simulink model "CSTR_mpc8_simulink"  (R2023b)
settings: Solver=VariableStepAuto  StartTime=0.0  StopTime=10.0  RelTol=1e-3
libraries: mpclib x1, cstblocks x1
settings Model: Creator=epepe  LastModifiedBy=epepe

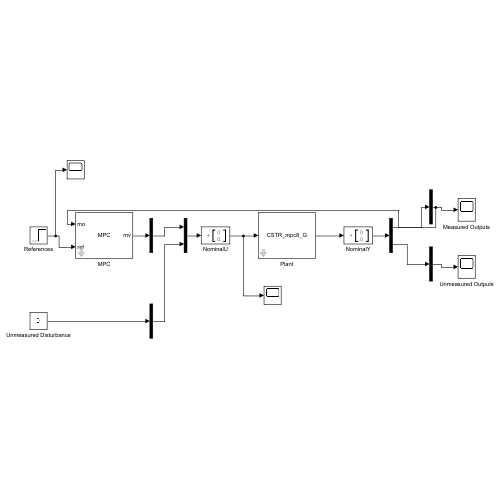
[thumbnail: Simulink's stored preview of the top-level diagram]
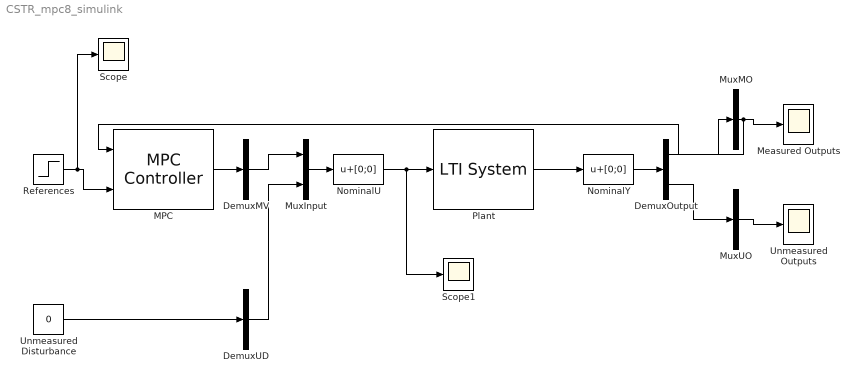
== system CSTR_mpc8_simulink ==
  DemuxMV : Demux  Outputs=1
  DemuxOutput : Demux  Outputs=2
  DemuxUD : Demux  Outputs=1
  MPC : mpclib/MPC Controller  SCDEnableBlockLinearizationSpecification=on  mpcobj=CSTR_mpc8_C  is_multiple=0  enable_value=0  return_u0=off  updateMPCinCallerWorkspace=on  md_inport=off  mv_inport=off  uref_inport=off  return_cost=off  return_mvseq=off  return_qpstatus=off  return_xseq=off  return_state=off  return_ovseq=off  state_inport=off  umin_inport=off  umax_inport=off  ymin_inport=off  ymax_inport=off  cc_inport=off  ywt_inport=off  uwt_inport=off  duwt_inport=off  rhoeps_inport=off  pm_inport=off  MaximumP=10  HorizonChoice=FixedHorizon  n_ts=0.5  n_p=15  n_mv=1  n_md=0  n_ud=1  n_mo=1  n_uo=1  BlockDataType=double  SampleTimeInherited=off  switch_inport=off
  Measured Outputs : Scope
  MuxInput : Mux  Inputs=2
  MuxMO : Mux  Inputs=1
  MuxUO : Mux  Inputs=1
  NominalU : Bias  Bias=[0;0]
  NominalY : Bias  Bias=[0;0]
  Plant : cstblocks/LTI System  sys=CSTR_mpc8_G  IC=[]  PadeOrder=0
  References : Step  Time=5  Before=[0;0]  After=[2;0]
  Scope : Scope
  Scope1 : Scope
  Unmeasured Disturbance : Constant  Value=0
  Unmeasured Outputs : Scope
  wires:
  References/1 -> Scope/1, MPC/2
  Plant/1 -> NominalY/1
  NominalY/1 -> DemuxOutput/1
  MuxMO/1 -> MPC/1, Measured Outputs/1
  MuxUO/1 -> Unmeasured Outputs/1
  DemuxOutput/1 -> MuxMO/1
  DemuxOutput/2 -> MuxUO/1
  MuxInput/1 -> NominalU/1
  NominalU/1 -> Scope1/1, Plant/1
  MPC/1 -> DemuxMV/1
  DemuxMV/1 -> MuxInput/1
  Unmeasured Disturbance/1 -> DemuxUD/1
  DemuxUD/1 -> MuxInput/2
